simulink subsystem "power_window_system_impact_V6"  (R2021a)
settings: Solver=VariableStepAuto  StartTime=0.0  StopTime=10.0  RelTol=1e-3
libraries: BCM x4
settings Model: Creator=achu  LastModifiedBy=Sai229

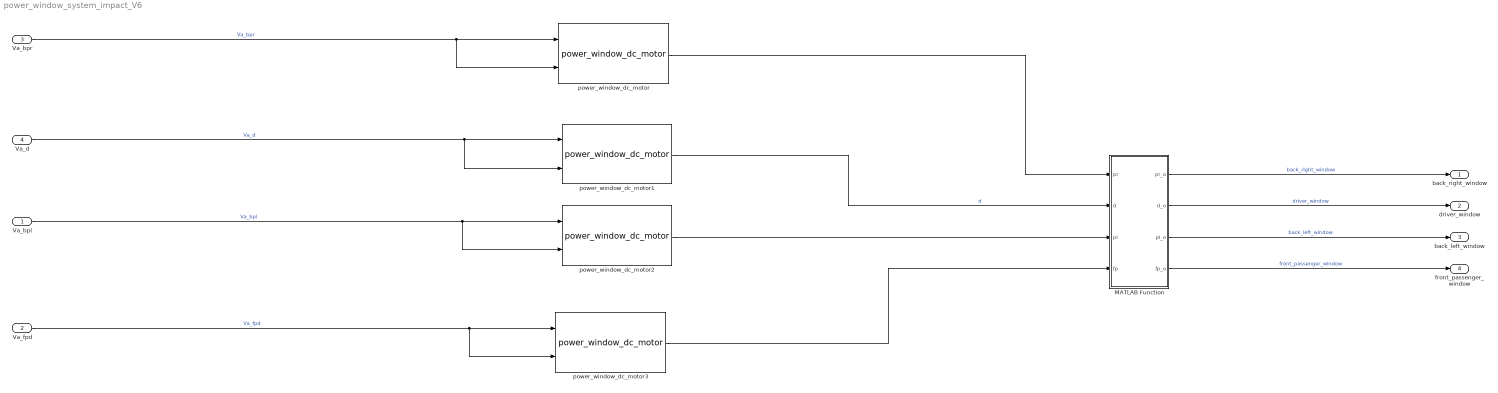
== system power_window_system_impact_V6 ==
  Va_bpl : Inport
  Va_fpd : Inport  Port=2
  Va_bpr : Inport  Port=3
  Va_d : Inport  Port=4
  MATLAB Function : MATLAB Function  TreatAsAtomicUnit=on
  power_window_dc_motor{,1..3} (4 alike) : BCM/power_window_dc_motor  SystemSampleTime=-1  VariantActivationTime=update diagram  Latency=0  AutoFrameSizeCalculation=off
      settings: SourceProductName=BCM Library
  back_right_window : Outport
  driver_window : Outport  Port=2
  back_left_window : Outport  Port=3
  front_passenger_window : Outport  Port=4
  wires:
  Va_fpd/1 -> power_window_dc_motor3/1, power_window_dc_motor3/2  "Va_fpd"
  Va_d/1 -> power_window_dc_motor1/1, power_window_dc_motor1/2  "Va_d"
  power_window_dc_motor3/1 -> MATLAB Function/4(fp)
  power_window_dc_motor2/1 -> MATLAB Function/3(pl)
  power_window_dc_motor1/1 -> MATLAB Function/2(d)  "d"
  MATLAB Function/1(pr_o) -> back_right_window/1  "back_right_window"
  power_window_dc_motor/1 -> MATLAB Function/1(pr)
  Va_bpr/1 -> power_window_dc_motor/1, power_window_dc_motor/2  "Va_bpr"
  Va_bpl/1 -> power_window_dc_motor2/1, power_window_dc_motor2/2  "Va_bpl"
  MATLAB Function/2(d_o) -> driver_window/1  "driver_window"
  MATLAB Function/3(pl_o) -> back_left_window/1  "back_left_window"
  MATLAB Function/4(fp_o) -> front_passenger_window/1  "front_passenger_window"

== matlab function power_window_system_impact_V6/MATLAB Function ==
  data: pr input; pr_o output; d input; pl input; fp input; d_o output; pl_o output; fp_o output
function [pr_o,d_o, pl_o, fp_o] = fcn(pr, d, pl, fp)
if pr>=10
    prout=10;
elseif pr<=0
    prout=0;
else
    prout=pr;
end

if d>=10
    dout=10;
elseif d<=0
    dout=0;
else
    dout=d;
end

if pl>=10
    plout=10;
elseif pl<=0
    plout=0;
else
    plout=pr;
end

if fp>=10
    fpout=10;
elseif fp<=0
    fpout=0;
else
    fpout=fp;
end
pr_o=prout;
d_o=dout;
pl_o=plout;
fp_o=fpout;
